simulink model "TRAMI_DCT_AT"  (R2018b)
settings: Solver=FixedStepDiscrete  StartTime=0.0  StopTime=88  FixedStep=10e-3  RelTol=1e-3  EnableMultiTasking=on
undefined symbols (not defined in the file): CONST_AP_GEAR_SUB_NEWTRAL, CONST_AP_IDLE_SPEED_CONT, CONST_AP_LOAD_SFT, CONST_AP_LOAD_SFT_HYS, CONST_CAR_WEIGHT, CONST_CL_NUM, CONST_F_DOWN_SYNCHRO, CONST_F_SYNCHRO, CONST_F_UP_SYNCHRO, CONST_FGR, CONST_I_FlYWHEEL, CONST_INATIA_CLANK, CONST_R_SHIFT_END_CD, CONST_R_SHIFT_END_EG, CONST_R_SHIFT_END_TD, CONST_R_SHIFT_END_UP, CONST_R_SYNCHRO_ENGAGE, CONST_R_TIRE, CONST_RATIO_TQ_REDUCTION, CONST_SKIP_SHIFT_MAX, CONST_SYN_NUM, CONST_T_SFT_END_EN, CONST_T_SFT_END_JUDGE, CONST_T_SFT_END_MAX, CONST_T_SFT_END_MIN, CONST_T_SHIFT_WAIT, CONST_T_TQ_PHASE_CD, CONST_T_TQ_PHASE_ND, CONST_T_TQ_PHASE_NR, CONST_T_TQ_PHASE_TD, CONST_T_TQ_PHASE_UP, CONST_TQ_CREEP_CONT, CONST_TQ_ENGAGE_CL_MARGIN, CONST_TQ_ENGAGE_CL_MIN, CONST_TQ_INATIA_TD_SHIFT, CONST_TQ_LOAD_SFT, CONST_TQ_LOAD_SFT_HYS, CONST_TQ_ND_ENGAGE, CONST_TQ_NR_ENGAGE, CONST_TQ_TQPHASE_MIN, CONST_V_IDLE_SPEED_CONT, Eng, FALSE, GrNP, GrRev, LoopTime, MAT_CL_ENGAGE, MAT_CL_SHARE_RATE, MAT_I_ACTUATOR, MAT_SYNCHRO_COM, MAT_T_GEAR_SUB_NEWTRAL, MAT_TRANS_MGR, MaxCL, Nm, PI, Shift_CD, Shift_ND, Shift_NR, Shift_TD, Shift_Up ... (+168)
libraries: simulink x26
(part 2 of 6)

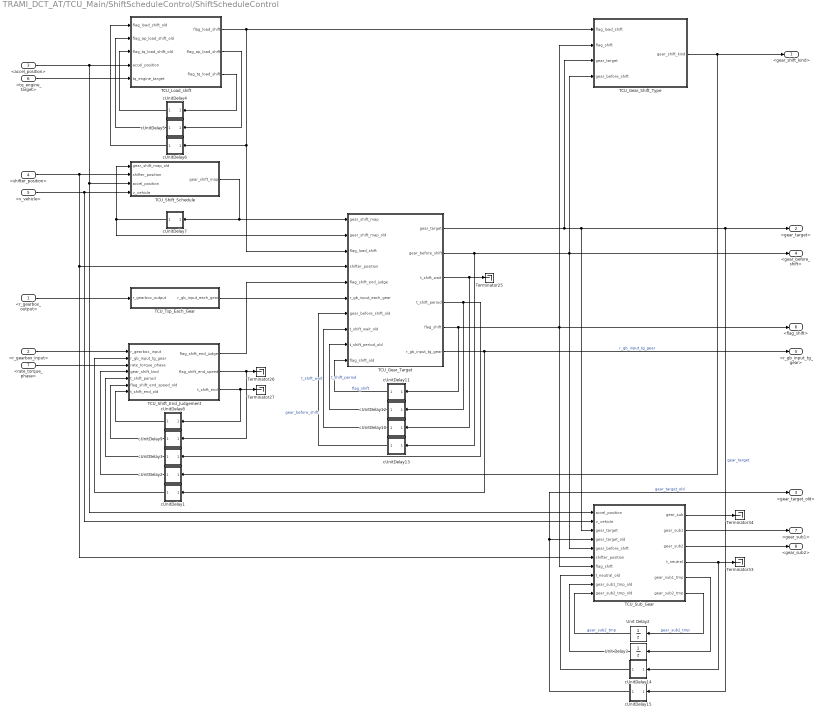
== system TRAMI_DCT_AT/TCU_Main/ShiftScheduleControl/ShiftScheduleControl ==
  <r_gearbox_output> : Inport  OutDataTypeStr=single
  <r_gearbox_input> : Inport  Port=2  OutDataTypeStr=single
  <accel_position> : Inport  Port=3  OutDataTypeStr=single
  <shifter_position> : Inport  Port=4  OutDataTypeStr=int16
  <v_vehicle> : Inport  Port=5  OutDataTypeStr=single
  <tq_engine_target> : Inport  Port=6  OutDataTypeStr=single
  <rate_torque_phase> : Inport  Port=7  OutDataTypeStr=single
  TCU_Gear_Shift_Type : Subsystem
      settings: AttributesFormatString=変速種別判定
  TCU_Gear_Target : Subsystem
      settings: AttributesFormatString=目標ギヤ段の決定
  TCU_Load_shift : Subsystem
      settings: AttributesFormatString=駆動・被駆動判定
  TCU_Shift_End_Judgement : Subsystem
      settings: AttributesFormatString=変速終了判定
  TCU_Shift_Schedule : Subsystem
      settings: AttributesFormatString=マップで定められたギヤ段の算出
  TCU_Sub_Gear : Subsystem
      settings: AttributesFormatString=DCTの待機ギヤ段の決定
  TCU_Tsp_Each_Gear : Subsystem
      settings: AttributesFormatString=各ギヤ段でのGearBox入力回転の演算
  Terminator{25..27,33..34} (5 alike) : Terminator
  Unit Delay2 : UnitDelay  SampleTime=-1
  Unit Delay3 : UnitDelay  SampleTime=-1
  cUnitDelay1 : Subsystem  mask(resetable_unit_delay){initParam=0}
      mask prompts: initParam "初期化値"
      mask Display:
      | dpoly(1,[1,0],'z')
      | text(2,10,'R')
  cUnitDelay10 : Subsystem  mask(resetable_unit_delay){initParam=0}
      mask prompts: initParam "初期化値"
      mask Display:
      | dpoly(1,[1,0],'z')
      | text(2,10,'R')
  cUnitDelay11 : Subsystem  mask(resetable_unit_delay){initParam=0}
      mask prompts: initParam "初期化値"
      mask Display:
      | dpoly(1,[1,0],'z')
      | text(2,10,'R')
  cUnitDelay12 : Subsystem  mask(resetable_unit_delay){initParam=0}
      mask prompts: initParam "初期化値"
      mask Display:
      | dpoly(1,[1,0],'z')
      | text(2,10,'R')
  cUnitDelay13 : Subsystem  mask(resetable_unit_delay){initParam=0}
      mask prompts: initParam "初期化値"
      mask Display:
      | dpoly(1,[1,0],'z')
      | text(2,10,'R')
  cUnitDelay14 : Subsystem  mask(resetable_unit_delay){initParam=0}
      mask prompts: initParam "初期化値"
      mask Display:
      | dpoly(1,[1,0],'z')
      | text(2,10,'R')
  cUnitDelay15 : Subsystem  mask(resetable_unit_delay){initParam=0}
      mask prompts: initParam "初期化値"
      mask Display:
      | dpoly(1,[1,0],'z')
      | text(2,10,'R')
  cUnitDelay2 : Subsystem  mask(resetable_unit_delay){initParam=0}
      mask prompts: initParam "初期化値"
      mask Display:
      | dpoly(1,[1,0],'z')
      | text(2,10,'R')
  cUnitDelay3 : Subsystem  mask(resetable_unit_delay){initParam=0}
      mask prompts: initParam "初期化値"
      mask Display:
      | dpoly(1,[1,0],'z')
      | text(2,10,'R')
  cUnitDelay4 : Subsystem  mask(resetable_unit_delay){initParam=0}
      mask prompts: initParam "初期化値"
      mask Display:
      | dpoly(1,[1,0],'z')
      | text(2,10,'R')
  cUnitDelay5 : Subsystem  mask(resetable_unit_delay){initParam=0}
      mask prompts: initParam "初期化値"
      mask Display:
      | dpoly(1,[1,0],'z')
      | text(2,10,'R')
  cUnitDelay6 : Subsystem  mask(resetable_unit_delay){initParam=0}
      mask prompts: initParam "初期化値"
      mask Display:
      | dpoly(1,[1,0],'z')
      | text(2,10,'R')
  cUnitDelay7 : Subsystem  mask(resetable_unit_delay){initParam=0}
      mask prompts: initParam "初期化値"
      mask Display:
      | dpoly(1,[1,0],'z')
      | text(2,10,'R')
  cUnitDelay8 : Subsystem  mask(resetable_unit_delay){initParam=0}
      mask prompts: initParam "初期化値"
      mask Display:
      | dpoly(1,[1,0],'z')
      | text(2,10,'R')
  cUnitDelay9 : Subsystem  mask(resetable_unit_delay){initParam=0}
      mask prompts: initParam "初期化値"
      mask Display:
      | dpoly(1,[1,0],'z')
      | text(2,10,'R')
  <gear_shift_kind> : Outport  OutDataTypeStr=int16
  <gear_target> : Outport  Port=2  OutDataTypeStr=int16
  <gear_target_old> : Outport  Port=3  OutDataTypeStr=int16
  <gear_before_shift> : Outport  Port=4  OutDataTypeStr=int16
  <r_gb_input_tg_gear> : Outport  Port=5  OutDataTypeStr=single
  <flag_shift> : Outport  Port=6  OutDataTypeStr=boolean
  <gear_sub1> : Outport  Port=7  OutDataTypeStr=int16
  <gear_sub2> : Outport  Port=8  OutDataTypeStr=int16
  wires:
  TCU_Sub_Gear/4(t_neutral) -> cUnitDelay14/1(<param>), Terminator33/1
  TCU_Gear_Target/5(flag_shift) -> TCU_Gear_Shift_Type/2(flag_shift), <flag_shift>/1, TCU_Sub_Gear/7(flag_shift), cUnitDelay11/1(<param>)
  cUnitDelay1/1(preParam) -> TCU_Shift_End_Judgement/2(r_gb_input_tg_gear)
  TCU_Gear_Target/1(gear_target) -> TCU_Gear_Shift_Type/3(gear_target), <gear_target>/1, cUnitDelay15/1(<param>), TCU_Sub_Gear/3(gear_target)  "gear_target"
  <accel_position>/1 -> TCU_Sub_Gear/1(accel_position), TCU_Shift_Schedule/3(accel_position), TCU_Load_shift/4(accel_position)
  TCU_Gear_Target/3(t_shift_wait) -> cUnitDelay10/1(<param>), Terminator25/1
  TCU_Sub_Gear/2(gear_sub1) -> <gear_sub1>/1
  TCU_Shift_End_Judgement/3(t_shift_end) -> cUnitDelay8/1(<param>), Terminator27/1
  cUnitDelay2/1(preParam) -> TCU_Shift_End_Judgement/4(gear_shift_kind)
  TCU_Load_shift/2(flag_ap_load_shift) -> cUnitDelay5/1(<param>)
  TCU_Load_shift/1(flag_load_shift) -> cUnitDelay6/1(<param>), TCU_Gear_Target/3(flag_load_shift), TCU_Gear_Shift_Type/1(flag_load_shift)
  TCU_Shift_End_Judgement/1(flag_shift_end_judge) -> TCU_Gear_Target/5(flag_shift_end_judge)
  cUnitDelay15/1(preParam) -> <gear_target_old>/1, TCU_Sub_Gear/4(gear_target_old)  "gear_target_old"
  TCU_Gear_Target/6(r_gb_input_tg_gear) -> <r_gb_input_tg_gear>/1, cUnitDelay1/1(<param>)  "r_gb_input_tg_gear"
  TCU_Gear_Shift_Type/1(gear_shift_kind) -> <gear_shift_kind>/1, cUnitDelay2/1(<param>)
  cUnitDelay3/1(preParam) -> TCU_Shift_End_Judgement/5(t_shift_period)
  TCU_Sub_Gear/1(gear_sub) -> Terminator34/1
  TCU_Load_shift/3(flag_tq_load_shift) -> cUnitDelay4/1(<param>)
  TCU_Shift_End_Judgement/2(flag_shift_end_speed) -> Terminator26/1, cUnitDelay9/1(<param>)
  TCU_Tsp_Each_Gear/1(r_gb_input_each_gear) -> TCU_Gear_Target/6(r_gb_input_each_gear)
  <v_vehicle>/1 -> TCU_Shift_Schedule/4(v_vehicle), TCU_Sub_Gear/2(v_vehicle)
  TCU_Shift_Schedule/1(gear_shift_map) -> TCU_Gear_Target/1(gear_shift_map), cUnitDelay7/1(<param>)
  <r_gearbox_input>/1 -> TCU_Shift_End_Judgement/1(r_gearbox_input)
  <rate_torque_phase>/1 -> TCU_Shift_End_Judgement/3(rate_torque_phase)
  <tq_engine_target>/1 -> TCU_Load_shift/5(tq_engine_target)
  <r_gearbox_output>/1 -> TCU_Tsp_Each_Gear/1(r_gearbox_output)
  <shifter_position>/1 -> TCU_Shift_Schedule/2(shifter_position), TCU_Sub_Gear/6(shifter_position), TCU_Gear_Target/4(shifter_position)
  cUnitDelay4/1(preParam) -> TCU_Load_shift/3(flag_tq_load_shift_old)
  cUnitDelay5/1(preParam) -> TCU_Load_shift/2(flag_ap_load_shift_old)
  cUnitDelay6/1(preParam) -> TCU_Load_shift/1(flag_load_shift_old)
  cUnitDelay7/1(preParam) -> TCU_Gear_Target/2(gear_shift_map_old), TCU_Shift_Schedule/1(gear_shift_map_old)
  cUnitDelay8/1(preParam) -> TCU_Shift_End_Judgement/7(t_shift_end_old)
  cUnitDelay9/1(preParam) -> TCU_Shift_End_Judgement/6(flag_shift_end_speed_old)
  cUnitDelay10/1(preParam) -> TCU_Gear_Target/8("  t_shift_wait_old")  "t_shift_wait"
  cUnitDelay11/1(preParam) -> TCU_Gear_Target/10("  flag_shift_old")  "flag_shift"
  TCU_Gear_Target/4(t_shift_period) -> cUnitDelay12/1(<param>), cUnitDelay3/1(<param>)
  cUnitDelay12/1(preParam) -> TCU_Gear_Target/9("  t_shift_period_old")  "t_shift_period"
  TCU_Gear_Target/2(gear_before_shift) -> cUnitDelay13/1(<param>), TCU_Sub_Gear/5(gear_before_shift), <gear_before_shift>/1, TCU_Gear_Shift_Type/4(gear_before_shift)
  cUnitDelay13/1(preParam) -> TCU_Gear_Target/7("  gear_before_shift_old")  "gear_before_shift"
  TCU_Sub_Gear/6(gear_sub2_tmp) -> Unit Delay2/1  "gear_sub2_tmp"
  Unit Delay2/1 -> TCU_Sub_Gear/10(gear_sub2_tmp_old)  "gear_sub2_tmp"
  TCU_Sub_Gear/5(gear_sub1_tmp) -> Unit Delay3/1
  Unit Delay3/1 -> TCU_Sub_Gear/9(gear_sub1_tmp_old)
  TCU_Sub_Gear/3(gear_sub2) -> <gear_sub2>/1
  cUnitDelay14/1(preParam) -> TCU_Sub_Gear/8(t_neutral_old)

== system TRAMI_DCT_AT/TCU_Main/StartingDeviceControl/StartingDeviceControl ==
  <r_gearbox_input> : Inport  OutDataTypeStr=single
  <accel_position> : Inport  Port=2  OutDataTypeStr=single
  <v_vehicle> : Inport  Port=3  OutDataTypeStr=single
  <r_engine> : Inport  Port=4  OutDataTypeStr=single
  <tq_engine_target> : Inport  Port=5  OutDataTypeStr=single
  <r_engine_idle> : Inport  Port=6  OutDataTypeStr=single
  <gear_ratio> : Inport  Port=7  OutDataTypeStr=single
  <gear_target> : Inport  Port=8  OutDataTypeStr=int16
  <r_gb_input_tg_gear> : Inport  Port=9  OutDataTypeStr=single
  <gear_target_old> : Inport  Port=10  OutDataTypeStr=int16
  <flag_shift> : Inport  Port=11  OutDataTypeStr=boolean
  TCU_Creep_Control : Subsystem
      settings: AttributesFormatString=クリープトルク制御
  TCU_Engin_Idle_Control : Subsystem
      settings: AttributesFormatString=Engineによるアイドル回転制御の実行判定
  TCU_Fluid_Coupling_Torque : Subsystem
      settings: AttributesFormatString=トルクコンバータ特性の演算
  TCU_Slip_Control : Subsystem
      settings: AttributesFormatString=発進デバイスのスリップ制御
  TCU_Torque_Input_GearBox : Subsystem
      settings: AttributesFormatString=GearBox入力トルクの算出
  Terminator{1,4..6,21..22,35..37} (9 alike) : Terminator
  <tq_cl_creep_cont> : Outport  OutDataTypeStr=single
  <tq_torq_converter_input> : Outport  Port=2  OutDataTypeStr=single
  <tq_gearbox_input> : Outport  Port=3  OutDataTypeStr=single
  <tq_cl_slip_control> : Outport  Port=4  OutDataTypeStr=single
  <tq_cl_slip_base> : Outport  Port=5  OutDataTypeStr=single
  flag_engine_idle_control : Outport  Port=6  OutDataTypeStr=boolean
  wires:
  TCU_Fluid_Coupling_Torque/4(torq_ratio_torq_converter) -> TCU_Torque_Input_GearBox/2(torq_ratio_torq_converter)
  <tq_engine_target>/1 -> TCU_Slip_Control/4(tq_engine_target), TCU_Torque_Input_GearBox/1(tq_engine_target)
  TCU_Slip_Control/2(r_cl_slip_target) -> Terminator22/1
  TCU_Creep_Control/1(tq_cl_creep_cont) -> <tq_cl_creep_cont>/1
  <r_engine>/1 -> TCU_Slip_Control/2(r_engine), TCU_Fluid_Coupling_Torque/1(r_engine)
  TCU_Slip_Control/3(r_cl_slip_act) -> Terminator21/1
  TCU_Slip_Control/6(tq_cl_slip_base) -> <tq_cl_slip_base>/1
  TCU_Fluid_Coupling_Torque/1(tq_torq_converter_input) -> <tq_torq_converter_input>/1
  TCU_Slip_Control/5(tq_torq_converter_slip_tg) -> Terminator37/1
  TCU_Slip_Control/4(r_engine_slip_target) -> Terminator36/1
  TCU_Slip_Control/8(tq_flyweel_output) -> Terminator35/1
  <flag_shift>/1 -> TCU_Slip_Control/1(flag_shift)  "flag_shift"
  <r_gb_input_tg_gear>/1 -> TCU_Slip_Control/3(r_gb_input_tg_gear), TCU_Engin_Idle_Control/5(<r_gb_input_tg_gear>)  "r_gb_input_tg_gear"
  TCU_Torque_Input_GearBox/1(tq_gearbox_input) -> <tq_gearbox_input>/1
  TCU_Fluid_Coupling_Torque/2(tq_torq_converter_output) -> Terminator4/1
  TCU_Fluid_Coupling_Torque/5(cap_factor_torq_converter) -> Terminator6/1
  TCU_Fluid_Coupling_Torque/3(spd_ratio_torq_converter) -> Terminator5/1
  TCU_Slip_Control/1(tq_cl_slip_control) -> <tq_cl_slip_control>/1
  <gear_target_old>/1 -> TCU_Slip_Control/8(gear_target_old)  "gear_target_old"
  <r_engine_idle>/1 -> TCU_Engin_Idle_Control/1(<r_engine_idle>), TCU_Slip_Control/5(r_engine_idle)  "r_engine_idle"
  <gear_target>/1 -> TCU_Engin_Idle_Control/4(<gear_target>), TCU_Slip_Control/7(gear_target), TCU_Creep_Control/1(gear_target)  "gear_target"
  <r_gearbox_input>/1 -> TCU_Fluid_Coupling_Torque/2(r_gearbox_input)
  TCU_Slip_Control/7(tq_cl_slip_correct) -> Terminator1/1
  <gear_ratio>/1 -> TCU_Slip_Control/6(gear_ratio)  "gear_ratio"
  <accel_position>/1 -> TCU_Engin_Idle_Control/2(<accel_position>)
  <v_vehicle>/1 -> TCU_Engin_Idle_Control/3(<v_vehicle>)
  TCU_Engin_Idle_Control/1(<flag_engine_idle_control>) -> flag_engine_idle_control/1, TCU_Slip_Control/9(flag_engine_idle_control)

== system TRAMI_DCT_AT/TCU_Main/AccControl/AccControl/TCU_Acutuator_Control ==
  gear_target : Inport  OutDataTypeStr=int16
      settings: AttributesFormatString=目標ギヤ段[-]
  Constant : Constant  Value=MAT_I_ACTUATOR  OutDataTypeStr=single
  Selector : Selector  IndexMode=Zero-based  InputPortWidth=12  IndexOptions=Index vector (port)  Indices=[1 3]  OutputSizes=1
  i_actuator : Outport  OutDataTypeStr=single
      settings: AttributesFormatString=アクチュエータ消費電流[A]
  wires:
  Constant/1 -> Selector/1
  gear_target/1 -> Selector/2
  Selector/1 -> i_actuator/1  "i_actuator"

== system TRAMI_DCT_AT/TCU_Main/AccControl/AccControl/TCU_Cooler_Flow_Rate_Control ==
  temp_trans_fluid : Inport  OutDataTypeStr=single
      settings: AttributesFormatString=トランスミッション油温[℃]
  Table_search_2D1 : Lookup_n-D  NumberOfTableDimensions=1  BreakpointsForDimension1=T2D_Q_TRANS_FLUID_X  Table=T2D_Q_TRANS_FLUID_Y  ExtrapMethod=Clip  UseLastTableValue=on  InternalRulePriority=Speed  OutDataTypeStr=single  RndMeth=Simplest  InputSameDT=on
      settings: AttributesFormatString=|
      | tbl = %<Table>
      | axis = %<BreakpointsForDimension1>
  Table_search_2D2 : Lookup_n-D  NumberOfTableDimensions=1  BreakpointsForDimension1=T2D_Q_ENGINE_WATER_X  Table=T2D_Q_ENGINE_WATER_Y  ExtrapMethod=Clip  UseLastTableValue=on  InternalRulePriority=Speed  OutDataTypeStr=single  RndMeth=Simplest  InputSameDT=on
      settings: AttributesFormatString=|
      | tbl = %<Table>
      | axis = %<BreakpointsForDimension1>
  q_cooler_trans_fluid : Outport  OutDataTypeStr=single
      settings: AttributesFormatString=トランスミッションオイル流量[L/min]
  q_cooler_engine_water : Outport  Port=2  OutDataTypeStr=single
      settings: AttributesFormatString=冷却水量[L/min]
  wires:
  Table_search_2D1/1 -> q_cooler_trans_fluid/1  "q_cooler_trans_fluid"
  Table_search_2D2/1 -> q_cooler_engine_water/1  "q_cooler_engine_water"
  temp_trans_fluid/1 -> Table_search_2D1/1, Table_search_2D2/1

== system TRAMI_DCT_AT/TCU_Main/AccControl/AccControl/TCU_EOP_Control ==
  temp_trans_fluid : Inport  OutDataTypeStr=single
      settings: AttributesFormatString=トランスミッション油温[℃]
  r_engine : Inport  Port=2  OutDataTypeStr=single
      settings: AttributesFormatString=エンジン回転数[rpm]
  Table_search_3D_sample6 : Subsystem  mask(Table_search_3D){map=T3D_I_EOP, tbl_x=T2DX_I_EOP_Y, axis_x=T2DX_I_EOP_X, tbl_y=T2DY_I_EOP_Y, axis_y=T2DY_I_EOP_X}
      mask Display:
      | disp('Table_search_3D');
      | 
      | port_label('input',  1, 'X' );
      | port_label('input',  2, 'Y' );
      | port_label('output', 1, 'out' );
  i_eop : Outport  OutDataTypeStr=single
      settings: AttributesFormatString=EOP電流[A]
  wires:
  r_engine/1 -> Table_search_3D_sample6/1(X)
  temp_trans_fluid/1 -> Table_search_3D_sample6/2(Y)
  Table_search_3D_sample6/1(out) -> i_eop/1  "i_eop"

== system TRAMI_DCT_AT/TCU_Main/AccControl/AccControl/TCU_Pressure_Line_Control ==
  tq_gearbox_input : Inport  OutDataTypeStr=single
      settings: AttributesFormatString=GearBox入力トルク[Nm]
  gear_target : Inport  Port=2  OutDataTypeStr=int16
      settings: AttributesFormatString=目標ギヤ段[-]
  Constant : Constant  Value=T2D_P_LINE_Y  OutDataTypeStr=single
  Constant1 : Constant  Value=T2D_P_LINE_X  OutDataTypeStr=single
  Lookup Table Dynamic : simulink/Lookup Tables/Lookup Table Dynamic  LookUpMeth=Interpolation-Use End Values  OutDataType=fixdt('single')  OutScaling=[]  OutputDataTypeScalingMode=Specify via dialog  OutDataTypeStr=fixdt('single')  DoSatur=off
      settings: SourceProductName=Simulink
  Selector : Selector  NumberOfDimensions=2  IndexMode=Zero-based  InputPortWidth=3  IndexOptions=Index vector (port),Select all  Indices=[1 3],1  OutputSizes=1,1
  Selector1 : Selector  NumberOfDimensions=2  IndexMode=Zero-based  InputPortWidth=3  IndexOptions=Index vector (port),Select all  Indices=[1 3],1  OutputSizes=1,1
  p_line : Outport  OutDataTypeStr=single
      settings: AttributesFormatString=ライン圧[kPa]
  wires:
  tq_gearbox_input/1 -> Lookup Table Dynamic/1
  Lookup Table Dynamic/1 -> p_line/1  "p_line"
  Selector/1 -> Lookup Table Dynamic/3
  Selector1/1 -> Lookup Table Dynamic/2
  Constant/1 -> Selector/1
  Constant1/1 -> Selector1/1
  gear_target/1 -> Selector1/2, Selector/2

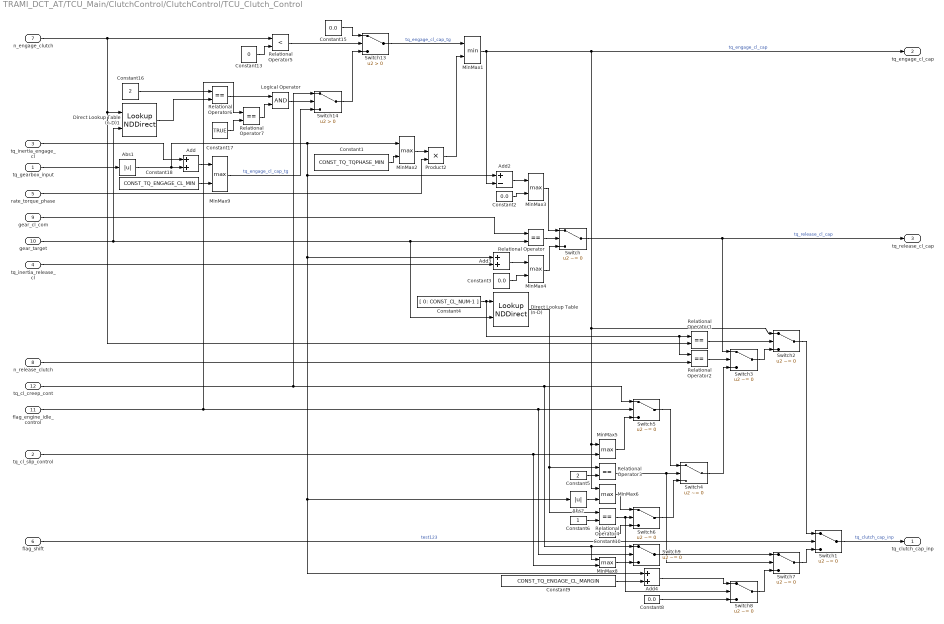
== system TRAMI_DCT_AT/TCU_Main/ClutchControl/ClutchControl/TCU_Clutch_Control ==
  tq_gearbox_input : Inport  OutDataTypeStr=single
      settings: AttributesFormatString=GearBox入力トルク[Nm]
  tq_cl_slip_control : Inport  Port=2  OutDataTypeStr=single
      settings: AttributesFormatString=スリップ制御クラッチのトルク容量[Nm]
  tq_inertia_engage_cl : Inport  Port=3  OutDataTypeStr=single
      settings: AttributesFormatString=締結クラッチのイナーシャトルク[Nm]
  tq_inertia_release_cl : Inport  Port=4  OutDataTypeStr=single
      settings: AttributesFormatString=解放クラッチのイナーシャトルク[Nm]
  rate_torque_phase : Inport  Port=5  OutDataTypeStr=single
      settings: AttributesFormatString=トルクフェイズ移行比率[-]
  flag_shift : Inport  Port=6  OutDataTypeStr=boolean
      settings: AttributesFormatString=シフトフラグ[-]
  n_engage_clutch : Inport  Port=7  OutDataTypeStr=int16
      settings: AttributesFormatString=締結クラッチ[-]
  n_release_clutch : Inport  Port=8  OutDataTypeStr=int16
      settings: AttributesFormatString=解放クラッチ[-]
  gear_cl_com : Inport  Port=9  OutDataTypeStr=int16
      settings: AttributesFormatString=Clutch制御用ギヤ段[-]
  gear_target : Inport  Port=10  OutDataTypeStr=int16
      settings: AttributesFormatString=目標ギヤ段[-]
  flag_engine_idle_control : Inport  Port=11  OutDataTypeStr=boolean
      settings: AttributesFormatString=|
      | アイドル回転制御の実行判定フラグ
      | TRUE ：Engによるアイドル回転制御を実行
      | FALSE：クラッチスリップ制御によるEng回転制御を行う
      | [-]
  tq_cl_creep_cont : Inport  Port=12  OutDataTypeStr=single
      settings: AttributesFormatString=クリープ制御のためのクラッチトルク容量[Nm]
  Abs1 : Abs  OutDataTypeStr=single
  Abs2 : Abs  OutDataTypeStr=single
  Add : Sum  AccumDataTypeStr=single  OutDataTypeStr=single
  Add2 : Sum  Inputs=+-  OutDataTypeStr=single
  Add3 : Sum  OutDataTypeStr=single
  Add4 : Sum  OutDataTypeStr=single
  Constant1 : Constant  Value=CONST_TQ_TQPHASE_MIN  OutDataTypeStr=int16
  Constant{2..3,8,10,15} (5 alike) : Constant  Value=0.0  OutDataTypeStr=single
  Constant13 : Constant  Value=0  OutDataTypeStr=int16
  Constant16 : Constant  Value=2  OutDataTypeStr=int16
  Constant17 : Constant  Value=TRUE  OutDataTypeStr=boolean
  Constant18 : Constant  Value=CONST_TQ_ENGAGE_CL_MIN  OutDataTypeStr=single
  Constant4 : Constant  Value=[ 0: CONST_CL_NUM-1 ]  OutDataTypeStr=int16
  Constant5 : Constant  Value=2  OutDataTypeStr=int16
  Constant6 : Constant  OutDataTypeStr=int16
  Constant9 : Constant  Value=CONST_TQ_ENGAGE_CL_MARGIN  OutDataTypeStr=single
  Direct Lookup Table (n-D) : LookupNDDirect  Table=MAT_CL_ENGAGE  TableDataTypeStr=int16
  Direct Lookup Table (n-D)1 : LookupNDDirect  Table=MAT_CL_ENGAGE  TableDataTypeStr=int16
  Logical Operator : Logic  AllPortsSameDT=off  OutDataTypeStr=boolean
  MinMax1 : MinMax  Inputs=2  OutDataTypeStr=single
  MinMax{2..6,8..9} (7 alike) : MinMax  Function=max  Inputs=2  OutDataTypeStr=single
  Product2 : Product  OutDataTypeStr=single
  Relational Operator{,1..4} (5 alike) : RelationalOperator  Operator===  OutDataTypeStr=boolean  RndMeth=Nearest
  Relational Operator5 : RelationalOperator  Operator=<  OutDataTypeStr=boolean  RndMeth=Simplest
  Relational Operator6 : RelationalOperator  Operator===  OutDataTypeStr=boolean  RndMeth=Simplest
  Relational Operator7 : RelationalOperator  Operator===  OutDataTypeStr=boolean  RndMeth=Simplest
  Switch{,1..9} (10 alike) : Switch  Criteria=u2 ~= 0  OutDataTypeStr=single
  Switch13 : Switch  Criteria=u2 > Threshold  OutDataTypeStr=single
  Switch14 : Switch  Criteria=u2 > Threshold  OutDataTypeStr=single
  tq_clutch_cap_inp : Outport  OutDataTypeStr=single
      settings: AttributesFormatString=各クラッチのトルク容量[Nm]
  tq_engage_cl_cap : Outport  Port=2  OutDataTypeStr=single
      settings: AttributesFormatString=締結クラッチトルク容量[Nm]
  tq_release_cl_cap : Outport  Port=3  OutDataTypeStr=single
      settings: AttributesFormatString=開放クラッチトルク容量[Nm]
  wires:
  Constant9/1 -> Add4/2
  Add4/1 -> Switch8/1
  Switch/1 -> tq_release_cl_cap/1, Switch3/1  "tq_release_cl_cap"
  Switch1/1 -> tq_clutch_cap_inp/1  "tq_clutch_cap_inp"
  MinMax4/1 -> Switch/3
  MinMax6/1 -> Switch6/1
  tq_inertia_engage_cl/1 -> Add/1
  Abs2/1 -> MinMax6/2
  Switch7/1 -> Switch1/3
  gear_cl_com/1 -> Relational Operator/1
  MinMax5/1 -> Switch5/3
  Relational Operator/1 -> Switch/2
  Switch6/1 -> Switch4/3
  Relational Operator2/1 -> Switch3/2
  Constant6/1 -> Relational Operator4/2
  tq_cl_slip_control/1 -> MinMax5/2, MinMax8/2
  Switch5/1 -> Switch4/1
  tq_inertia_release_cl/1 -> Add3/2
  Constant5/1 -> Relational Operator3/2
  n_release_clutch/1 -> Relational Operator2/2
  Abs1/1 -> Add3/1, Abs2/1, Add4/1, Add2/1, MinMax2/1, Add/2
  Switch3/1 -> Switch2/3
  MinMax3/1 -> Switch/1
  Direct Lookup Table (n-D)/1 -> Relational Operator3/1, Relational Operator4/1
  tq_gearbox_input/1 -> Abs1/1
  Switch2/1 -> Switch1/1
  gear_target/1 -> Relational Operator/2, Direct Lookup Table (n-D)/2, Direct Lookup Table (n-D)1/2
  MinMax1/1 -> Add2/2, MinMax6/1, MinMax5/1, Switch2/1, tq_engage_cl_cap/1  "tq_engage_cl_cap"
  Constant3/1 -> MinMax4/2
  Relational Operator1/1 -> Switch2/2
  n_engage_clutch/1 -> Relational Operator1/2, Direct Lookup Table (n-D)1/1, Relational Operator5/1
  flag_shift/1 -> Switch1/2  "test123"
  Constant4/1 -> Relational Operator2/1, Relational Operator1/1, Direct Lookup Table (n-D)/1
  Switch8/1 -> Switch7/3
  Add3/1 -> MinMax4/1
  Add2/1 -> MinMax3/1
  rate_torque_phase/1 -> Product2/2
  Constant2/1 -> MinMax3/2
  Constant8/1 -> Switch8/3
  Relational Operator3/1 -> Switch4/2, Switch7/2
  Relational Operator4/1 -> Switch8/2, Switch6/2
  Switch9/1 -> Switch7/1
  flag_engine_idle_control/1 -> Relational Operator7/1, Switch5/2, Switch9/2
  tq_cl_creep_cont/1 -> Switch14/1, Switch9/1, MinMax8/1, Switch5/1
  MinMax8/1 -> Switch9/3
  Constant10/1 -> Switch6/3
  Relational Operator5/1 -> Switch13/2
  Constant13/1 -> Relational Operator5/2
  Constant15/1 -> Switch13/1
  Switch14/1 -> Switch13/3
  Direct Lookup Table (n-D)1/1 -> Relational Operator6/2
  Constant16/1 -> Relational Operator6/1
  Relational Operator6/1 -> Logical Operator/1
  Relational Operator7/1 -> Logical Operator/2
  Constant17/1 -> Relational Operator7/2
  Logical Operator/1 -> Switch14/2
  Add/1 -> MinMax9/1
  Constant18/1 -> MinMax9/2
  MinMax9/1 -> Switch14/3  "tq_engage_cl_cap_tg"
  Switch13/1 -> MinMax1/1  "tq_engage_cl_cap_tg"
  MinMax2/1 -> Product2/1
  Constant1/1 -> MinMax2/2
  Product2/1 -> MinMax1/2
  Switch4/1 -> Switch3/3

== system TRAMI_DCT_AT/TCU_Main/ClutchControl/ClutchControl/TCU_Clutch_Torque_Capacity ==
  gear_target : Inport  OutDataTypeStr=int16
      settings: AttributesFormatString=目標ギヤ段[-]
  gear_before_shift : Inport  Port=2  OutDataTypeStr=int16
      settings: AttributesFormatString=変速前ギヤ段[-]
  tq_clutch_cap_inp : Inport  Port=3  OutDataTypeStr=single
      settings: AttributesFormatString=各クラッチのトルク容量[Nm]
  Constant : Constant  Value=[ 0:CONST_CL_NUM-1 ]  OutDataTypeStr=int16
  Direct Lookup Table (n-D) : LookupNDDirect  Table=MAT_CL_SHARE_RATE  TableDataTypeStr=single
  Direct Lookup Table (n-D)1 : LookupNDDirect  Table=MAT_CL_SHARE_RATE  TableDataTypeStr=single
  MinMax : MinMax  Function=max  Inputs=2  OutDataTypeStr=single
  Product : Product  OutDataTypeStr=single
  tq_clutch_cap : Outport  OutDataTypeStr=single
      settings: AttributesFormatString=クラッチのトルク容量[Nm]
  rate_clutch_share : Outport  Port=2  OutDataTypeStr=single
      settings: AttributesFormatString=分担トルク[-]
  wires:
  Product/1 -> tq_clutch_cap/1  "tq_clutch_cap"
  gear_before_shift/1 -> Direct Lookup Table (n-D)1/2
  Direct Lookup Table (n-D)/1 -> MinMax/1
  Direct Lookup Table (n-D)1/1 -> MinMax/2
  Constant/1 -> Direct Lookup Table (n-D)1/1, Direct Lookup Table (n-D)/1
  gear_target/1 -> Direct Lookup Table (n-D)/2
  tq_clutch_cap_inp/1 -> Product/2
  MinMax/1 -> rate_clutch_share/1, Product/1  "rate_clutch_share"

== system TRAMI_DCT_AT/TCU_Main/ClutchControl/ClutchControl/TCU_Gear_Clutch_Control ==
  flag_synchro_ready : Inport  OutDataTypeStr=boolean
      settings: AttributesFormatString=シンクロの同期判定[-]
  gear_target : Inport  Port=2  OutDataTypeStr=int16
      settings: AttributesFormatString=目標ギヤ段[-]
  gear_before_shift : Inport  Port=3  OutDataTypeStr=int16
      settings: AttributesFormatString=変速前ギヤ段[-]
  gear_shift_kind : Inport  Port=4  OutDataTypeStr=int16
      settings: AttributesFormatString=|
      | ギヤ変速種別
      | 5 : N->R
      | 4 : N->D
      | 3 : Torque demand shift
      | 2 : Coast down shift
      | 1 : Schedule up shift
      | [-]
  r_gearbox_input : Inport  Port=5  OutDataTypeStr=single
      settings: AttributesFormatString=Gearbox input speed[rpm]
  r_gb_input_tg_gear : Inport  Port=6  OutDataTypeStr=single
      settings: AttributesFormatString=|
      | 目標ギヤ段でのGearBox入力回転
      | （GearBox出力回転から演算)[rpm]
  Constant : Constant  Value=FALSE  OutDataTypeStr=boolean
  Constant1 : Constant  Value=GrRev  OutDataTypeStr=int16
  Constant2 : Constant  Value=Shift_TD  OutDataTypeStr=int16
  Logical Operator : Logic  Operator=OR  AllPortsSameDT=off  OutDataTypeStr=boolean
  Relational Operator{1..4} (4 alike) : RelationalOperator  Operator===  OutDataTypeStr=boolean  RndMeth=Nearest
  Relational Operator5 : RelationalOperator  OutDataTypeStr=boolean  RndMeth=Nearest
  Switch{1..4} (4 alike) : Switch  Criteria=u2 ~= 0  OutDataTypeStr=int16
  cUnitDelay2 : Subsystem  mask(resetable_unit_delay){initParam=0}
      mask prompts: initParam "初期化値"
      mask Display:
      | dpoly(1,[1,0],'z')
      | text(2,10,'R')
  gear_cl_com : Outport  OutDataTypeStr=int16
      settings: AttributesFormatString=Clutch制御用ギヤ段[-]
  wires:
  cUnitDelay2/1(preParam) -> Switch3/1, Switch4/3  "gear_cl_com"
  Relational Operator2/1 -> Switch3/2
  Switch1/1 -> Switch3/3
  flag_synchro_ready/1 -> Relational Operator2/1  "flag_synchro_ready"
  Constant/1 -> Relational Operator2/2
  Logical Operator/1 -> Switch1/2
  Relational Operator3/1 -> Logical Operator/2
  Relational Operator1/1 -> Logical Operator/1
  Switch2/1 -> Switch1/3
  Constant1/1 -> Relational Operator3/2, Relational Operator1/2
  gear_before_shift/1 -> Relational Operator3/1  "gear_before_shift"
  Relational Operator4/1 -> Switch2/2
  gear_shift_kind/1 -> Relational Operator4/1
  Constant2/1 -> Relational Operator4/2
  Switch4/1 -> Switch2/1
  Relational Operator5/1 -> Switch4/2
  r_gearbox_input/1 -> Relational Operator5/1
  r_gb_input_tg_gear/1 -> Relational Operator5/2
  gear_target/1 -> Relational Operator1/1, Switch1/1, Switch2/3, Switch4/1  "gear_target"
  Switch3/1 -> cUnitDelay2/1(<param>), gear_cl_com/1  "gear_cl_com"

== system TRAMI_DCT_AT/TCU_Main/ClutchControl/ClutchControl/TCU_SYNCHORO_CONTROL_AT_DCT ==
  note: 1) Add Subsystem or Model blocks as valid variant choices.
      | 2) You cannot connect blocks at this level. At simulation, connectivity is automatically
      | determined, based on the active variant and port name matching.
  gear_target : Inport  OutDataTypeStr=int16
  gear_before_shift : Inport  Port=2  OutDataTypeStr=int16
  gear_sub1 : Inport  Port=3  OutDataTypeStr=int16
  gear_sub2 : Inport  Port=4  OutDataTypeStr=int16
  f_synchro_old : Inport  Port=5  OutDataTypeStr=single
  TCU_SYNCHORO_CONTROL_AT : Subsystem  VariantControl=CONST_SYN_NUM == 0
  TCU_SYNCHORO_CONTROL_DCT : Subsystem  VariantControl=CONST_SYN_NUM > 0
  f_synchro : Outport  OutDataTypeStr=single
  flag_synchro_com : Outport  Port=2  OutDataTypeStr=boolean

== system TRAMI_DCT_AT/TCU_Main/ClutchControl/ClutchControl/TCU_SYNCHORO_STATUS_AT_DCT ==
  note: 1) Add Subsystem or Model blocks as valid variant choices.
      | 2) You cannot connect blocks at this level. At simulation, connectivity is automatically
      | determined, based on the active variant and port name matching.
  gear_target : Inport  OutDataTypeStr=int16
      settings: AttributesFormatString=目標ギヤ段[-]
  f_synchro : Inport  Port=2  OutDataTypeStr=single
      settings: AttributesFormatString=シンクロの押し力[N]
  r_synchoro_dif : Inport  Port=3  OutDataTypeStr=single
      settings: AttributesFormatString=各シンクロ差回転[rpm]
  TCU_SYNCHORO_STATUS_AT : Subsystem  VariantControl=CONST_SYN_NUM == 0
  TCU_SYNCHORO_STATUS_DCT : Subsystem  VariantControl=CONST_SYN_NUM > 0
  flag_synchro_ready : Outport  OutDataTypeStr=boolean
      settings: AttributesFormatString=全シンクロの同期判定[-]

== system TRAMI_DCT_AT/TCU_Main/ClutchControl/ClutchControl/TCU_Shift_Clutch ==
  gear_target : Inport  OutDataTypeStr=int16
      settings: AttributesFormatString=目標ギヤ段[-]
  gear_before_shift : Inport  Port=2  OutDataTypeStr=int16
      settings: AttributesFormatString=変速前ギヤ段[-]
  Bias1 : Bias  Bias=-1
  Bias2 : Bias  Bias=-1
  Compare To Constant : simulink/Logic and Bit Operations/Compare To Constant  relop=>  const=0  OutDataTypeStr=boolean
  Compare To Constant1 : simulink/Logic and Bit Operations/Compare To Constant  relop===  const=0  OutDataTypeStr=boolean
  Compare To Constant2 : simulink/Logic and Bit Operations/Compare To Constant  relop===  const=0  OutDataTypeStr=boolean
  Compare To Constant3 : simulink/Logic and Bit Operations/Compare To Constant  relop=>  const=0  OutDataTypeStr=boolean
  Constant : Constant  Value=[0:MaxCL-1]  OutDataTypeStr=single
  Constant1 : Constant  Value=[0:MaxCL-1]  OutDataTypeStr=single
  Constant2 : Constant  Value=1:MaxCL  OutDataTypeStr=int16
  Constant4 : Constant  Value=1:MaxCL  OutDataTypeStr=int16
  Direct Lookup Table (n-D){,1..3} (4 alike) : LookupNDDirect  Table=MAT_CL_ENGAGE
  Logical Operator : Logic  AllPortsSameDT=off  OutDataTypeStr=boolean
  Logical Operator1 : Logic  AllPortsSameDT=off  OutDataTypeStr=boolean
  MinMax1 : MinMax  Function=max  OutDataTypeStr=int16
  MinMax2 : MinMax  Function=max  OutDataTypeStr=int16
  Product1 : Product  OutDataTypeStr=int16
  Product2 : Product  OutDataTypeStr=int16
  n_engage_clutch : Outport  OutDataTypeStr=int16
      settings: AttributesFormatString=締結クラッチ[-]
  n_release_clutch : Outport  Port=2  OutDataTypeStr=int16
      settings: AttributesFormatString=解放クラッチ[-]
  wires:
  Constant/1 -> Direct Lookup Table (n-D)1/1, Direct Lookup Table (n-D)/1
  Compare To Constant/1 -> Logical Operator/1
  Compare To Constant1/1 -> Logical Operator/2
  Direct Lookup Table (n-D)1/1 -> Compare To Constant1/1
  Direct Lookup Table (n-D)/1 -> Compare To Constant/1
  Direct Lookup Table (n-D)2/1 -> Compare To Constant2/1
  gear_before_shift/1 -> Direct Lookup Table (n-D)2/2, Direct Lookup Table (n-D)/2  "gear_before_shift"
  gear_target/1 -> Direct Lookup Table (n-D)1/2, Direct Lookup Table (n-D)3/2  "gear_target"
  Direct Lookup Table (n-D)3/1 -> Compare To Constant3/1
  Compare To Constant3/1 -> Logical Operator1/2
  Compare To Constant2/1 -> Logical Operator1/1
  Constant1/1 -> Direct Lookup Table (n-D)2/1, Direct Lookup Table (n-D)3/1
  Logical Operator1/1 -> Product1/1
  Bias2/1 -> n_engage_clutch/1  "n_engage_clutch"
  Product1/1 -> MinMax1/1
  Constant4/1 -> Product1/2
  MinMax1/1 -> Bias2/1
  MinMax2/1 -> Bias1/1
  Constant2/1 -> Product2/2
  Product2/1 -> MinMax2/1
  Bias1/1 -> n_release_clutch/1  "n_release_clutch"
  Logical Operator/1 -> Product2/1

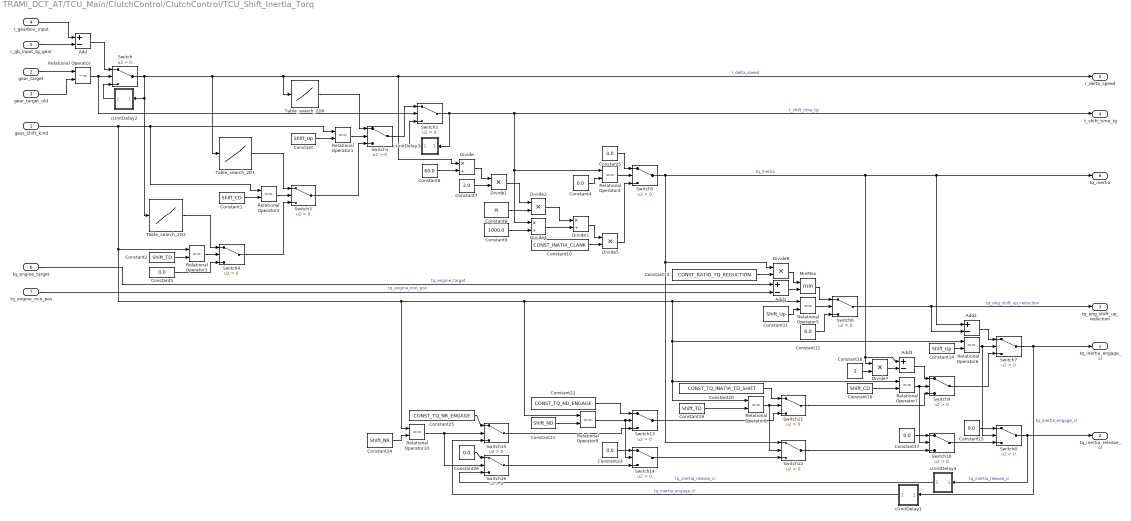
== system TRAMI_DCT_AT/TCU_Main/ClutchControl/ClutchControl/TCU_Shift_Inertia_Torq ==
  gear_shift_kind : Inport  OutDataTypeStr=int16
      settings: AttributesFormatString=|
      | ギヤ変速種別
      | 5 : N->R
      | 4 : N->D
      | 3 : Torque demand shift
      | 2 : Coast down shift
      | 1 : Schedule up shift
      | [-]
  gear_target : Inport  Port=2  OutDataTypeStr=int16
      settings: AttributesFormatString=目標ギヤ段[-]
  gear_target_old : Inport  Port=3  OutDataTypeStr=int16
      settings: AttributesFormatString=前回の目標ギヤ段[-]
  r_gearbox_input : Inport  Port=4  OutDataTypeStr=single
      settings: AttributesFormatString=Gearbox input speed[rpm]
  r_gb_input_tg_gear : Inport  Port=5  OutDataTypeStr=single
      settings: AttributesFormatString=|
      | 目標ギヤ段でのGearBox入力回転
      | （GearBox出力回転から演算)[rpm]
  tq_engine_target : Inport  Port=6  OutDataTypeStr=single
      settings: AttributesFormatString=目標エンジントルク[Nm]
  tq_engine_min_pos : Inport  Port=7  OutDataTypeStr=single
      settings: AttributesFormatString=Eng.出力可能最小トルク[Nm]
  Add{,1..3} (4 alike) : Sum  Inputs=+-  OutDataTypeStr=single
  Constant : Constant  Value=Shift_Up  OutDataTypeStr=int16
  Constant1 : Constant  Value=Shift_CD  OutDataTypeStr=int16
  Constant10 : Constant  Value=CONST_INATIA_CLANK  OutDataTypeStr=single
  Constant11 : Constant  Value=Shift_Up  OutDataTypeStr=int16
  Constant{3..5,12,15,17,23,26} (8 alike) : Constant  Value=0.0  OutDataTypeStr=single
  Constant13 : Constant  Value=CONST_RATIO_TQ_REDUCTION  OutDataTypeStr=single
  Constant14 : Constant  Value=Shift_Up  OutDataTypeStr=int16
  Constant16 : Constant  Value=Shift_CD  OutDataTypeStr=int16
  Constant18 : Constant  Value=2  OutDataTypeStr=int16
  Constant19 : Constant  Value=Shift_TD  OutDataTypeStr=int16
  Constant2 : Constant  Value=Shift_TD  OutDataTypeStr=int16
  Constant20 : Constant  Value=CONST_TQ_INATIA_TD_SHIFT  OutDataTypeStr=single
  Constant21 : Constant  Value=Shift_ND  OutDataTypeStr=int16
  Constant22 : Constant  Value=CONST_TQ_ND_ENGAGE  OutDataTypeStr=single
  Constant24 : Constant  Value=Shift_NR  OutDataTypeStr=int16
  Constant25 : Constant  Value=CONST_TQ_NR_ENGAGE  OutDataTypeStr=single
  Constant6 : Constant  Value=60.0  OutDataTypeStr=single
  Constant7 : Constant  Value=2.0  OutDataTypeStr=single
  Constant8 : Constant  Value=PI  OutDataTypeStr=single
  Constant9 : Constant  Value=1000.0  OutDataTypeStr=single
  Divide : Product  Inputs=*/  OutDataTypeStr=single
  Divide{1..2,5..7} (5 alike) : Product  Inputs=**  OutDataTypeStr=single
  Divide3 : Product  Inputs=*/  OutDataTypeStr=single
  Divide4 : Product  Inputs=*/  OutDataTypeStr=single
  MinMax : MinMax  Inputs=2  OutDataTypeStr=single
  Relational Operator : RelationalOperator  Operator=~=  OutDataTypeStr=boolean  RndMeth=Nearest
  Relational Operator{1..10} (10 alike) : RelationalOperator  Operator===  OutDataTypeStr=boolean  RndMeth=Nearest
  Switch{,1..16} (17 alike) : Switch  Criteria=u2 > Threshold  OutDataTypeStr=single
  Table_search_2D1 : Lookup_n-D  NumberOfTableDimensions=1  BreakpointsForDimension1=T2D_T_SHIFT_TIME_TG_CD_X  Table=T2D_T_SHIFT_TIME_TG_CD_Y  TableDataTypeStr=single  ExtrapMethod=Clip  UseLastTableValue=on  InternalRulePriority=Speed  OutDataTypeStr=single  RndMeth=Simplest  InputSameDT=on
      settings: AttributesFormatString=|
      | tbl = %<Table>
      | axis = %<BreakpointsForDimension1>
  Table_search_2D2 : Lookup_n-D  NumberOfTableDimensions=1  BreakpointsForDimension1=T2D_T_SHIFT_TIME_TG_TD_X  Table=T2D_T_SHIFT_TIME_TG_TD_Y  TableDataTypeStr=single  ExtrapMethod=Clip  UseLastTableValue=on  InternalRulePriority=Speed  OutDataTypeStr=single  RndMeth=Simplest  InputSameDT=on
      settings: AttributesFormatString=|
      | tbl = %<Table>
      | axis = %<BreakpointsForDimension1>
  Table_search_2D6 : Lookup_n-D  NumberOfTableDimensions=1  BreakpointsForDimension1=T2D_T_SHIFT_TIME_TG_UP_X  Table=T2D_T_SHIFT_TIME_TG_UP_Y  TableDataTypeStr=single  ExtrapMethod=Clip  UseLastTableValue=on  InternalRulePriority=Speed  OutDataTypeStr=single  RndMeth=Simplest  InputSameDT=on
      settings: AttributesFormatString=|
      | tbl = %<Table>
      | axis = %<BreakpointsForDimension1>
  cUnitDelay1 : Subsystem  mask(resetable_unit_delay){initParam=0}
      mask prompts: initParam "初期化値"
      mask Display:
      | dpoly(1,[1,0],'z')
      | text(2,10,'R')
  cUnitDelay2 : Subsystem  mask(resetable_unit_delay){initParam=0}
      mask prompts: initParam "初期化値"
      mask Display:
      | dpoly(1,[1,0],'z')
      | text(2,10,'R')
  cUnitDelay3 : Subsystem  mask(resetable_unit_delay){initParam=0}
      mask prompts: initParam "初期化値"
      mask Display:
      | dpoly(1,[1,0],'z')
      | text(2,10,'R')
  cUnitDelay4 : Subsystem  mask(resetable_unit_delay){initParam=0}
      mask prompts: initParam "初期化値"
      mask Display:
      | dpoly(1,[1,0],'z')
      | text(2,10,'R')
  tq_inertia_engage_cl : Outport  OutDataTypeStr=single
      settings: AttributesFormatString=締結クラッチのイナーシャトルク[Nm]
  tq_inertia_release_cl : Outport  Port=2  OutDataTypeStr=single
      settings: AttributesFormatString=解放クラッチのイナーシャトルク[Nm]
  tq_eng_shift_up_reduction : Outport  Port=3  OutDataTypeStr=single
      settings: AttributesFormatString=アップシフト時のエンジントルクリダクション量[Nm]
  t_shift_time_tg : Outport  Port=4  OutDataTypeStr=single
      settings: AttributesFormatString=目標変速時間[ms]
  r_delta_speed : Outport  Port=5  OutDataTypeStr=single
      settings: AttributesFormatString=変速前後差回転[rpm]
  tq_inertia : Outport  Port=6  OutDataTypeStr=single
      settings: AttributesFormatString=イナーシャトルク[Nm]
  wires:
  gear_target/1 -> Relational Operator/1
  gear_target_old/1 -> Relational Operator/2
  Relational Operator/1 -> Switch/2, Switch2/2
  Add/1 -> Switch/1
  Switch/1 -> r_delta_speed/1, Divide/1, Table_search_2D6/1, Table_search_2D1/1, Table_search_2D2/1, cUnitDelay2/1(<param>)  "r_delta_speed"
  cUnitDelay2/1(preParam) -> Switch/3
  r_gb_input_tg_gear/1 -> Add/2
  r_gearbox_input/1 -> Add/1
  Relational Operator1/1 -> Switch1/2
  Constant/1 -> Relational Operator1/2
  Table_search_2D6/1 -> Switch1/1
  Switch3/1 -> Switch1/3
  Switch4/1 -> Switch3/3
  Constant1/1 -> Relational Operator2/2
  Relational Operator2/1 -> Switch3/2
  Relational Operator3/1 -> Switch4/2
  Table_search_2D2/1 -> Switch4/1
  Constant3/1 -> Switch4/3
  Table_search_2D1/1 -> Switch3/1
  Switch2/1 -> t_shift_time_tg/1, Relational Operator4/1, Divide4/1, cUnitDelay3/1(<param>)  "t_shift_time_tg"
  Switch1/1 -> Switch2/1
  cUnitDelay3/1(preParam) -> Switch2/3
  Constant4/1 -> Relational Operator4/2
  Relational Operator4/1 -> Switch5/2
  Constant5/1 -> Switch5/1
  Divide5/1 -> Switch5/3
  Constant6/1 -> Divide/2
  Divide/1 -> Divide1/1
  Constant7/1 -> Divide1/2
  Divide1/1 -> Divide2/1
  Constant8/1 -> Divide2/2
  Divide2/1 -> Divide3/1
  Divide4/1 -> Divide3/2
  Constant9/1 -> Divide4/2
  Divide3/1 -> Divide5/1
  Constant10/1 -> Divide5/2
  Constant2/1 -> Relational Operator3/2
  Constant11/1 -> Relational Operator5/2
  Relational Operator5/1 -> Switch6/2
  Constant12/1 -> Switch6/3
  MinMax/1 -> Switch6/1
  Divide6/1 -> MinMax/1
  Add1/1 -> MinMax/2
  Constant13/1 -> Divide6/2
  tq_engine_target/1 -> Add1/1  "tq_engine_target"
  tq_engine_min_pos/1 -> Add1/2  "tq_engine_min_pos"
  Constant14/1 -> Relational Operator6/2
  Relational Operator6/1 -> Switch7/2, Switch8/2
  Add2/1 -> Switch7/1
  Switch9/1 -> Switch7/3
  Constant15/1 -> Switch8/1
  Switch10/1 -> Switch8/3
  Constant16/1 -> Relational Operator7/2
  Relational Operator7/1 -> Switch9/2, Switch10/2
  Add3/1 -> Switch9/1
  Switch11/1 -> Switch9/3
  Constant17/1 -> Switch10/1
  Switch12/1 -> Switch10/3
  Divide7/1 -> Add3/2
  Constant18/1 -> Divide7/2
  Constant19/1 -> Relational Operator8/2
  Constant20/1 -> Switch11/1
  Switch13/1 -> Switch11/3
  Switch14/1 -> Switch12/3
  Switch5/1 -> tq_inertia/1, Add2/1, Add3/1, Divide7/1, Divide6/1, Switch12/1  "tq_inertia"
  Relational Operator8/1 -> Switch11/2, Switch12/2
  Constant21/1 -> Relational Operator9/2
  gear_shift_kind/1 -> Relational Operator5/1, Relational Operator6/1, Relational Operator7/1, Relational Operator8/1, Relational Operator9/1, Relational Operator10/1, Relational Operator3/1, Relational Operator2/1, Relational Operator1/1
  Relational Operator9/1 -> Switch13/2, Switch14/2
  Constant22/1 -> Switch13/1
  Switch15/1 -> Switch13/3
  Constant23/1 -> Switch14/1
  Switch16/1 -> Switch14/3
  Constant24/1 -> Relational Operator10/2
  Constant25/1 -> Switch15/1
  Switch7/1 -> tq_inertia_engage_cl/1, cUnitDelay1/1(<param>)  "tq_inertia_engage_cl"
  Switch8/1 -> tq_inertia_release_cl/1, cUnitDelay4/1(<param>)  "tq_inertia_release_cl"
  Constant26/1 -> Switch16/1
  Relational Operator10/1 -> Switch16/2, Switch15/2
  cUnitDelay1/1(preParam) -> Switch15/3  "tq_inertia_engage_cl"
  cUnitDelay4/1(preParam) -> Switch16/3  "tq_inertia_release_cl"
  Switch6/1 -> tq_eng_shift_up_reduction/1, Add2/2  "tq_eng_shift_up_reduction"

== system TRAMI_DCT_AT/TCU_Main/ClutchControl/ClutchControl/TCU_Torque_Phase ==
  flag_shift : Inport  OutDataTypeStr=boolean
      settings: AttributesFormatString=シフトフラグ[-]
  gear_shift_kind : Inport  Port=2  OutDataTypeStr=int16
      settings: AttributesFormatString=|
      | ギヤ変速種別
      | 5 : N->R
      | 4 : N->D
      | 3 : Torque demand shift
      | 2 : Coast down shift
      | 1 : Schedule up shift
      | [-]
  gear_cl_com : Inport  Port=3  OutDataTypeStr=int16
      settings: AttributesFormatString=Clutch制御用ギヤ段[-]
  gear_target : Inport  Port=4  OutDataTypeStr=int16
      settings: AttributesFormatString=目標ギヤ段[-]
  t_tq_phase_old : Inport  Port=5  OutDataTypeStr=single
      settings: AttributesFormatString=前回のトルクフェイズ経過時間[ms]
  Add : Sum  OutDataTypeStr=single
  Constant : Constant  Value=Shift_ND  OutDataTypeStr=int16
  Constant1 : Constant  Value=CONST_T_TQ_PHASE_ND  OutDataTypeStr=int16
  Constant10 : Constant  Value=0.0  OutDataTypeStr=single
  Constant2 : Constant  Value=Shift_NR  OutDataTypeStr=int16
  Constant3 : Constant  Value=CONST_T_TQ_PHASE_NR  OutDataTypeStr=int16
  Constant4 : Constant  Value=Shift_Up  OutDataTypeStr=int16
  Constant5 : Constant  Value=CONST_T_TQ_PHASE_UP  OutDataTypeStr=int16
  Constant6 : Constant  Value=Shift_TD  OutDataTypeStr=int16
  Constant7 : Constant  Value=CONST_T_TQ_PHASE_TD  OutDataTypeStr=int16
  Constant8 : Constant  Value=CONST_T_TQ_PHASE_CD  OutDataTypeStr=int16
  Constant9 : Constant  Value=LoopTime  OutDataTypeStr=single
  Divide : Product  Inputs=*/  OutDataTypeStr=single
  Logical Operator : Logic  AllPortsSameDT=off  OutDataTypeStr=boolean
  Relational Operator{1..5} (5 alike) : RelationalOperator  Operator===  OutDataTypeStr=boolean  RndMeth=Nearest
  Switch{,1..3} (4 alike) : Switch  Criteria=u2 > Threshold  OutDataTypeStr=int16
  Switch4 : Switch  Criteria=u2 > Threshold  OutDataTypeStr=single
  rate_torque_phase : Outport  OutDataTypeStr=single
      settings: AttributesFormatString=トルクフェイズ移行比率[-]
  t_tq_phase : Outport  Port=2  OutDataTypeStr=single
      settings: AttributesFormatString=トルクフェイズ経過時間[ms]
  wires:
  Constant/1 -> Relational Operator2/2
  Relational Operator2/1 -> Switch/2
  Constant1/1 -> Switch/1
  Constant3/1 -> Switch1/1
  Relational Operator1/1 -> Switch1/2
  Constant2/1 -> Relational Operator1/2
  Switch1/1 -> Switch/3
  Constant4/1 -> Relational Operator3/2
  Relational Operator3/1 -> Switch2/2
  Constant5/1 -> Switch2/1
  Switch2/1 -> Switch1/3
  Constant7/1 -> Switch3/1
  Relational Operator4/1 -> Switch3/2
  Constant6/1 -> Relational Operator4/2
  gear_shift_kind/1 -> Relational Operator1/1, Relational Operator2/1, Relational Operator3/1, Relational Operator4/1  "gear_shift_kind"
  Switch3/1 -> Switch2/3
  Constant8/1 -> Switch3/3
  flag_shift/1 -> Logical Operator/1  "flag_shift"
  gear_cl_com/1 -> Relational Operator5/1
  gear_target/1 -> Relational Operator5/2
  Logical Operator/1 -> Switch4/2
  Constant9/1 -> Add/1
  Switch4/1 -> t_tq_phase/1, Divide/1  "t_tq_phase"
  Constant10/1 -> Switch4/3
  t_tq_phase_old/1 -> Add/2
  Add/1 -> Switch4/1
  Divide/1 -> rate_torque_phase/1  "rate_torque_phase"
  Switch/1 -> Divide/2
  Relational Operator5/1 -> Logical Operator/2

== system TRAMI_DCT_AT/TCU_Main/ClutchControl/ClutchControl/cUnitDelay1 ==
  <param> : Inport
  Constant13 : Constant  Value=initParam  OutDataTypeStr=single
  Switch12 : Switch  Criteria=u2 > Threshold
  Unit Delay2 : UnitDelay  InitialCondition=zeros(size(initParam))  SampleTime=-1
  preParam : Outport
  wires:
  Unit Delay2/1 -> Switch12/3
  Switch12/1 -> preParam/1
  [FlagInit] -> Switch12/2
  Constant13/1 -> Switch12/1
  <param>/1 -> Unit Delay2/1

== system TRAMI_DCT_AT/TCU_Main/ClutchControl/ClutchControl/cUnitDelay3 ==
  <param> : Inport
  Constant13 : Constant  Value=initParam  OutDataTypeStr=single
  Switch12 : Switch  Criteria=u2 > Threshold
  Unit Delay2 : UnitDelay  InitialCondition=zeros(size(initParam))  SampleTime=-1
  preParam : Outport
  wires:
  <param>/1 -> Unit Delay2/1
  Constant13/1 -> Switch12/1
  [FlagInit] -> Switch12/2
  Switch12/1 -> preParam/1
  Unit Delay2/1 -> Switch12/3

== system TRAMI_DCT_AT/TCU_Main/GearControl/GearControl/TCU_Engine_Torque_Request ==
  tq_shift_up_target : Inport  OutDataTypeStr=single
      settings: AttributesFormatString=アップシフト時のエンジントルク目標値[Nm]
  flag_shift_up_tq_request : Inport  Port=2  OutDataTypeStr=boolean
      settings: AttributesFormatString=アップシフト時のトルクリダクション実行フラグ[-]
  Constant : Constant  Value=TRUE  OutDataTypeStr=boolean
  Constant1 : Constant  Value=1000.0  OutDataTypeStr=single
  Constant2 : Constant  Value=-1000.0  OutDataTypeStr=single
  Constant3 : Constant  Value=-1000.0  OutDataTypeStr=single
  Relational Operator : RelationalOperator  Operator===  OutDataTypeStr=boolean  RndMeth=Nearest
  Switch : Switch  Criteria=u2 > Threshold  OutDataTypeStr=single
  tq_engine_max_req : Outport  OutDataTypeStr=single
      settings: AttributesFormatString=エンジントルク最大値要求[Nm]
  tq_engine_min_req : Outport  Port=2  OutDataTypeStr=single
      settings: AttributesFormatString=エンジントルク最小値要求[Nm]
  r_engine_target : Outport  Port=3  OutDataTypeStr=single
      settings: AttributesFormatString=エンジン回転要求[Rpm]
  wires:
  Relational Operator/1 -> Switch/2
  Constant/1 -> Relational Operator/2
  flag_shift_up_tq_request/1 -> Relational Operator/1
  tq_shift_up_target/1 -> Switch/1
  Switch/1 -> tq_engine_max_req/1  "tq_engine_max_req"
  Constant1/1 -> Switch/3
  Constant2/1 -> tq_engine_min_req/1  "tq_engine_min_req"
  Constant3/1 -> r_engine_target/1  "r_engine_target"

== system TRAMI_DCT_AT/TCU_Main/GearControl/GearControl/TCU_Information_For_ECU ==
  gear_target : Inport  OutDataTypeStr=int16
      settings: AttributesFormatString=目標ギヤ段[-]
  flag_engine_idle_control : Inport  Port=2  OutDataTypeStr=boolean
      settings: AttributesFormatString=|
      | アイドル回転制御の実行判定フラグ
      | TRUE ：Engによるアイドル回転制御を実行
      | FALSE：クラッチスリップ制御によるEng回転制御を行う
      | [-]
  tq_torq_converter_input : Inport  Port=3  OutDataTypeStr=single
      settings: AttributesFormatString=トルコン流体伝達トルク(入力）[Nm]
  tq_cl_creep_cont : Inport  Port=4  OutDataTypeStr=single
      settings: AttributesFormatString=クリープ制御のためのクラッチトルク容量[Nm]
  tq_cl_slip_base : Inport  Port=5  OutDataTypeStr=single
      settings: AttributesFormatString=スリップクラッチのトルク容量基準値[Nm]
  Add : Sum  OutDataTypeStr=single
  Add1 : Sum  OutDataTypeStr=single
  Constant : Constant  Value=0  OutDataTypeStr=int16
  Constant1 : Constant  Value=GrRev  OutDataTypeStr=int16
  Constant3 : Constant  Value=MAT_TRANS_MGR  OutDataTypeStr=single
  Relational Operator2 : RelationalOperator  Operator=<  OutDataTypeStr=boolean  RndMeth=Nearest
  Selector : Selector  IndexMode=Zero-based  InputPortWidth=12  IndexOptions=Index vector (port)  Indices=[1 3]  OutputSizes=1
  Selector1 : Selector  IndexMode=Zero-based  InputPortWidth=12  IndexOptions=Index vector (port)  Indices=[1 3]  OutputSizes=1
  Switch : Switch  Criteria=u2 > Threshold  OutDataTypeStr=single
  Switch1 : Switch  Criteria=u2 > Threshold  OutDataTypeStr=single
  tq_trans_input : Outport  OutDataTypeStr=single
      settings: AttributesFormatString=トランスミッション入力軸トルク[Nm]
  gear_ratio : Outport  Port=2  OutDataTypeStr=single
      settings: AttributesFormatString=ギヤ比[-]
  flag_lock_up : Outport  Port=3  OutDataTypeStr=boolean
      settings: AttributesFormatString=flag_lock_up[-]
  wires:
  Switch/1 -> tq_trans_input/1  "tq_trans_input"
  tq_cl_creep_cont/1 -> Add/2
  tq_torq_converter_input/1 -> Add/1, Add1/1
  Add/1 -> Switch/1
  tq_cl_slip_base/1 -> Add1/2
  Add1/1 -> Switch/3
  Constant/1 -> Relational Operator2/2
  Relational Operator2/1 -> Switch1/2
  Selector/1 -> Switch1/1
  Selector1/1 -> Switch1/3
  Switch1/1 -> gear_ratio/1  "gear_ratio"
  Constant1/1 -> Selector/2
  gear_target/1 -> Relational Operator2/1, Selector1/2
  Constant3/1 -> Selector1/1, Selector/1
  flag_engine_idle_control/1 -> Switch/2, flag_lock_up/1  "flag_lock_up"
